simulink model "Udan_SOC"  (R2017b)
settings: Solver=FixedStepAuto  StartTime=0.0  StopTime=1000  FixedStep=0.1  RelTol=1e-3
values from neighbouring files (symbols this model uses):
  DenominatorOfIntegratorFactor = 100.0    [SOC_Stateflow.sldd]
  SOC_CalcSohLKT = 1.0    [SOC_Stateflow.sldd]
  SOC_CalcSOHTempLimit = 70.0    [SOC_Stateflow.sldd]
  SOC_CapPerCycle = 100.0    [SOC_Stateflow.sldd]
  SOC_CapTemp_HLimit = 200.0    [SOC_Stateflow.sldd]
  SOC_CapTemp_LLimit = 0.0    [SOC_Stateflow.sldd]
  Soc_ConfigInfo = 0    [SOC_Stateflow.sldd]
  SOC_DchgEndCalib = 0.0    [SOC_Stateflow.sldd]
  SOC_DiffVoltMin = 10.0    [SOC_Stateflow.sldd]
  SOC_DSOCJumpMax = 500.0    [SOC_Stateflow.sldd]
  SOC_EfficientHighLimit = 250.0    [SOC_Stateflow.sldd]
  SOC_EfficientLowLimit = 40.0    [SOC_Stateflow.sldd]
  SOC_EmptyAus = 0.0    [SOC_Stateflow.sldd]
  SOC_EnableOcv = 1.0    [SOC_Stateflow.sldd]
  SOC_END_CALIB_STATE : value not decoded    [SOC_Stateflow.sldd]
  SOC_HighRealSoc = 95.0    [SOC_Stateflow.sldd]
  SOC_LKTSohCycles = 0.0 1.0 10.0 20.0 30.0 40.0 50.0 60.0 70.0 80.0 90.0 100.0 110.0 120.0 130.0 140.0 150.0 160.0 170.0 180.0 190.0 200.0 210.0 220.0 230.0 240.0 250.0 260.0 270.0 280.0 290.0 300.0 310.0 320.0 330.0 340.0 350.0 360.0 370.0 380.0 390.0 400.0 410.0 420.0 430.0 440.0 450.0 460.0 470.0 480.0 490.0 500.0 510.0 520.0 530.0 540.0 550.0 560.0 570.0 580.0 590.0 600.0 610.0 620.0 630.0 640.0 650.0 660.0 670.0    [SOC_Stateflow.sldd]
  SOC_LKTSohTable = 1000.0 991.0 989.0 992.0 993.0 995.0 994.0 993.0 1000.0 997.0 1002.0 1000.0 992.0 1000.0 989.0 992.0 989.0 994.0 989.0 993.0 994.0 994.0 994.0 993.0 991.0 991.0 992.0 993.0 991.0 985.0 985.0 985.0 979.0 975.0 978.0 984.0 982.0 974.0 975.0 972.0 972.0 975.0 977.0 977.0 974.0 971.0 973.0 971.0 966.0 968.0 965.0 959.0 957.0 956.0 957.0 954.0 955.0 951.0 954.0 951.0 942.0 942.0 940.0 942.0 947.0 949.0    [SOC_Stateflow.sldd]
  SOC_LowRealSoc = 5.0    [SOC_Stateflow.sldd]
  SOC_NominalCap_AmS = 576000000.0    [SOC_Stateflow.sldd]
  SOC_NominalVol = 4000.0    [SOC_Stateflow.sldd]
  SOC_OCVTemp_HLimit = 106.0    [SOC_Stateflow.sldd]
  SOC_OCVTemp_LLimit = 29.0    [SOC_Stateflow.sldd]
  SOC_ShortCalibDSoc = 1.0    [SOC_Stateflow.sldd]
  SOC_SOCResolution = 10000.0    [SOC_Stateflow.sldd]
  SOC_SohCalcCapPercent = 8.0    [SOC_Stateflow.sldd]
  SOC_SohCalcHighLimit = 60.0    [SOC_Stateflow.sldd]
  SOC_SohCalcLowLimit = 10.0    [SOC_Stateflow.sldd]
  SOC_SohCalcMidLimit = 30.0    [SOC_Stateflow.sldd]
  SOC_SOHResolution = 1000.0    [SOC_Stateflow.sldd]
  SOC_State = <binary blob, 1163 chars, not shown>    [SOC_Stateflow.sldd]
  SOC_TempCap_CapBuffer : value not decoded    [SOC_Stateflow.sldd]
  SOC_TempCap_TempBuffer : value not decoded    [SOC_Stateflow.sldd]
  SocOcvCalib_ConfigInfo = 0.0    [SOC_Stateflow.sldd]
  SocOcvCalib_SocBuffer1 : value not decoded    [SOC_Stateflow.sldd]
  SocOcvCalib_TempBuffer : value not decoded    [SOC_Stateflow.sldd]
  SocOcvCalib_VoltageBuffer1 = 3300.0 3303.0 3305.0 3307.0 3310.0 3311.0 3313.0 3314.0 3316.0 3317.0 3319.0 3320.0 3322.0 3323.0 3325.0 3322.0 3323.0 3325.0 3310.0 3313.0 3315.0 3317.0 3320.0 3321.0 3323.0 3324.0 3326.0 3327.0 3329.0 3330.0 3332.0 3333.0 3335.0 3332.0 3333.0 3335.0 3320.0 3323.0 3325.0 3327.0 3330.0 3331.0 3333.0 3334.0 3336.0 3337.0 3339.0 3340.0 3342.0 3343.0 3345.0 3342.0 3343.0 3345.0 3330.0 3333.0 3335.0 3    [SOC_Stateflow.sldd]
  SOHCalibCycle = 10.0    [SOC_Stateflow.sldd]
undefined symbols (not defined in the file or in its folder): DatetimeM_GetReturnType, ParameterM_EeepParaIndexType, Soc_CumuLativeTypeType, SOC_EgthTempChgValue, Soc_EnergyBuffer, SOC_FithTempChgValue, SOC_FstSlowTempChgValue, SOC_FstTempChgValue, SOC_FthTempChgValue, SOC_MaxCap_AmS, SOC_SethTempChgValue, SOC_SixTempChgValue, SOC_SndSlowTempChgValue, SOC_SndTempChgValue, SOC_TrdSlowTempChgValue, SOC_TrdTempChgValue, SocDiagCalib_NoCalibReasonType
libraries: simulink x138, hdlsllib x24, dspindex x4
(part 1 of 10)
settings Model: DataDictionary=SOC_Stateflow.sldd  Creator=Administrator  LastModifiedBy=Administrator
settings OptimizationCC: DefaultParameterBehavior=Inlined  UseDivisionForNetSlopeComputation=on  PassReuseOutputArgsAs=Individual arguments  LifeSpan=inf
settings DebuggingCC: SignalInfNanChecking=error  IntegerOverflowMsg=error  ParameterTunabilityLossMsg=error  AssertControl=DisableAll  SFExecutionAtInitializationDiag=none
settings HardwareCC: ProdBitPerInt=16  ProdBitPerPointer=16  ProdBitPerSizeT=16  ProdBitPerPtrDiffT=16  ProdLargestAtomicFloat=None  ProdEndianess=BigEndian  ProdWordSize=16  ProdHWDeviceType=Freescale->HC(S)12
settings SFSimCC: MATLABDynamicMemAlloc=off
settings RTWCC: SystemTargetFile=ert.tlc  GenCodeOnly=on  TemplateMakefile=ert_default_tmf  GenerateReport=on  CustomSourceCode=/*lint -e* -w0 */  CustomHeaderCode=/*lint -e* -w0 */  Toolchain=MinGW64 | gmake (64-bit Windows)  IncludeHyperlinkInReport=on  GenerateTraceInfo=on  GenerateTraceReport=on  GenerateTraceReportSl=on  GenerateTraceReportSf=on  GenerateTraceReportEml=on
settings CodeAppCC: ForceParamTrailComments=on  IgnoreCustomStorageClasses=off  OperatorAnnotations=on  SimulinkDataObjDesc=on  SFDataObjDesc=on  InsertBlockDesc=on  StateflowObjectComments=on
settings ERTTargetCC: TargetLangStandard=C99 (ISO)  UtilityFuncGeneration=Shared location  SupportNonFinite=off  SupportVariableSizeSignals=on  ParenthesesLevel=Maximum  CastingMode=Standards  InlinedParameterPlacement=NonHierarchical  ERTCustomFileTemplate=example_file_process.tlc  GlobalDataDefinition=InSeparateSourceFile  DataDefinitionFile=UDAN_SOCCalibdata.c  DataReferenceFile=UDAN_SOCCalibdata.h  EnableSignedLeftShifts=off  EnableSignedRightShifts=off
settings ConfigComp: DVMaxProcessTime=30000  DVTestSuiteOptimization=CombinedObjectives (Nonlinear Extended)  DVDetectActiveLogic=on  DVDetectFloatOverflow=off  DVSaveReport=on

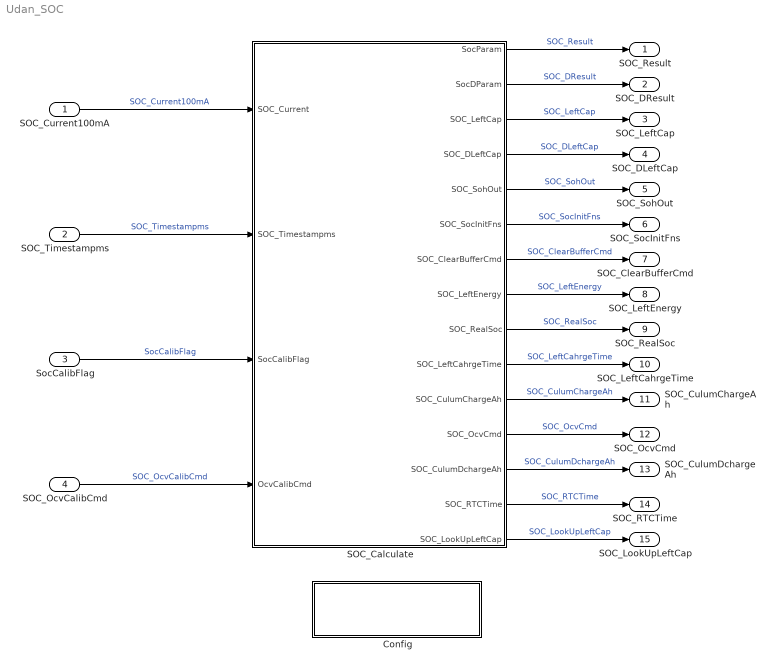
== system Udan_SOC ==
  SOC_Current100mA : Inport
  SOC_Timestampms : Inport  Port=2  OutDataTypeStr=uint32  PortDimensions=[1]
  SocCalibFlag : Inport  Port=3  OutDataTypeStr=uint8  PortDimensions=[1]
  SOC_OcvCalibCmd : Inport  Port=4
  Config : Subsystem
      mask help: 打开Ocv-Soc的电压曲线
      settings: OpenFcn=run('BlockConfig.m')
      mask Display: disp('双击完成Configuration配置')
  SOC_Calculate : Subsystem  TreatAsAtomicUnit=on  RTWFcnName=SOC_Calculate
      settings: RTWSystemCode=Nonreusable function  RTWFcnNameOpts=User specified
  SOC_Result : Outport
  SOC_DResult : Outport  Port=2
  SOC_LeftCap : Outport  Port=3
  SOC_DLeftCap : Outport  Port=4
  SOC_SohOut : Outport  Port=5
  SOC_SocInitFns : Outport  Port=6
  SOC_ClearBufferCmd : Outport  Port=7
  SOC_LeftEnergy : Outport  Port=8
  SOC_RealSoc : Outport  Port=9
  SOC_LeftCahrgeTime : Outport  Port=10
  SOC_CulumChargeAh : Outport  Port=11
  SOC_OcvCmd : Outport  Port=12
  SOC_CulumDchargeAh : Outport  Port=13
  SOC_RTCTime : Outport  Port=14
  SOC_LookUpLeftCap : Outport  Port=15
  wires:
  SOC_Calculate/1(SocParam) -> SOC_Result/1  "SOC_Result"
  SOC_Calculate/2(SocDParam) -> SOC_DResult/1  "SOC_DResult"
  SOC_Calculate/4(SOC_DLeftCap) -> SOC_DLeftCap/1  "SOC_DLeftCap"
  SOC_Calculate/3(SOC_LeftCap) -> SOC_LeftCap/1  "SOC_LeftCap"
  SOC_Current100mA/1 -> SOC_Calculate/1(SOC_Current)  "SOC_Current100mA"
  SOC_Calculate/5(SOC_SohOut) -> SOC_SohOut/1  "SOC_SohOut"
  SOC_Calculate/6(SOC_SocInitFns) -> SOC_SocInitFns/1  "SOC_SocInitFns"
  SOC_Timestampms/1 -> SOC_Calculate/2(SOC_Timestampms)  "SOC_Timestampms"
  SocCalibFlag/1 -> SOC_Calculate/3(SocCalibFlag)  "SocCalibFlag"
  SOC_Calculate/7(SOC_ClearBufferCmd) -> SOC_ClearBufferCmd/1  "SOC_ClearBufferCmd"
  SOC_Calculate/8(SOC_LeftEnergy) -> SOC_LeftEnergy/1  "SOC_LeftEnergy"
  SOC_Calculate/9(SOC_RealSoc) -> SOC_RealSoc/1  "SOC_RealSoc"
  SOC_Calculate/10(SOC_LeftCahrgeTime) -> SOC_LeftCahrgeTime/1  "SOC_LeftCahrgeTime"
  SOC_Calculate/11(SOC_CulumChargeAh) -> SOC_CulumChargeAh/1  "SOC_CulumChargeAh"
  SOC_Calculate/12(SOC_OcvCmd) -> SOC_OcvCmd/1  "SOC_OcvCmd"
  SOC_Calculate/13(SOC_CulumDchargeAh) -> SOC_CulumDchargeAh/1  "SOC_CulumDchargeAh"
  SOC_Calculate/14(SOC_RTCTime) -> SOC_RTCTime/1  "SOC_RTCTime"
  SOC_Calculate/15(SOC_LookUpLeftCap) -> SOC_LookUpLeftCap/1  "SOC_LookUpLeftCap"
  SOC_OcvCalibCmd/1 -> SOC_Calculate/4(OcvCalibCmd)  "SOC_OcvCalibCmd"

== system Udan_SOC/Config ==

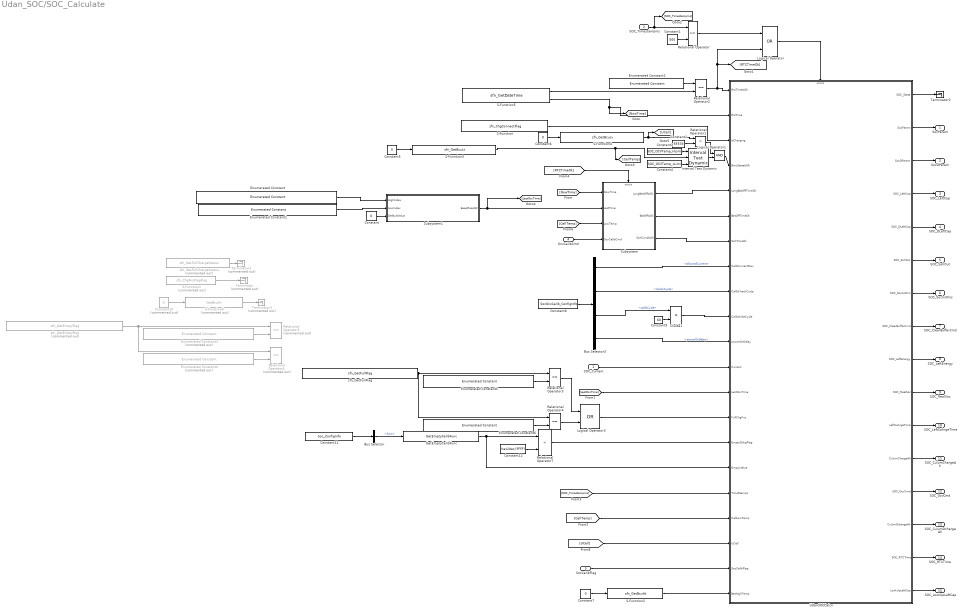
== system Udan_SOC/SOC_Calculate ==
  SOC_Current : Inport
  SOC_Timestampms : Inport  Port=2  OutDataTypeStr=uint32  PortDimensions=[1]
  SocCalibFlag : Inport  Port=3  OutDataTypeStr=uint8  PortDimensions=[1]
  OcvCalibCmd : Inport  Port=4
  Bus Selector : BusSelector  OutputSignals=func
  Bus Selector3 : BusSelector  OutputSignals=allowedCurrent,checkCycle,calibCycle,powerOnDelay
  Constant : Constant  Value=0  OutDataTypeStr=uint32
  Constant1 : Constant  Value=500  OutDataTypeStr=uint16
  Constant10 : Constant  Commented=on  Value=0  OutDataTypeStr=uint8
  Constant11 : Constant  Value=Soc_ConfigInfo  OutDataTypeStr=Bus: Soc_ConfigInfoType
  Constant12 : Constant  Value=hex2dec('FFFF')
  Constant2 : Constant  Value=65534  OutDataTypeStr=uint16
  Constant3 : Constant  Value=SOC_OCVTemp_HLimit  OutDataTypeStr=uint8
  Constant4 : Constant  Value=SOC_OCVTemp_LLimit  OutDataTypeStr=uint8
  Constant5 : Constant  Value=0  OutDataTypeStr=uint8
  Constant6 : Constant  Value=0  OutDataTypeStr=uint8
  Constant7 : Constant  Value=0  OutDataTypeStr=uint8
  Constant8 : Constant  Value=SocOcvCalib_ConfigInfo  OutDataTypeStr=Bus: SocOcvCalib_ConfigType
  Constant9 : Constant  Value=60  OutDataTypeStr=uint8
  Divide1 : Product  Inputs=**  OutDataTypeStr=uint32
  Enumerated Constant : simulink/Sources/Enumerated Constant  OutDataTypeStr=Enum: ParameterM_EeepParaIndexType  Value=ParameterM_EeepParaIndexType.PARAMETERM_EEEP_OCVSOC_TIME_HIGH_INDEX  SampleTime=inf
      settings: SourceProductName=Simulink
  Enumerated Constant1 : simulink/Sources/Enumerated Constant  OutDataTypeStr=Enum: ParameterM_EeepParaIndexType  Value=ParameterM_EeepParaIndexType.PARAMETERM_EEEP_OCVSOC_TIME_LOW_INDEX  SampleTime=inf
      settings: SourceProductName=Simulink
  Enumerated Constant2 : simulink/Sources/Enumerated Constant  OutDataTypeStr=Enum: DatetimeM_GetReturnType  Value=DatetimeM_GetReturnType.DATETIME_TRUSTY  SampleTime=inf
      settings: SourceProductName=Simulink
  Enumerated Constant3 : simulink/Sources/Enumerated Constant  Commented=on  OutDataTypeStr=Enum: SocDiagCalib_NoCalibReasonType  Value=SocDiagCalib_NoCalibReasonType.SOC_NO_CALIB_REASON_NORMAL  SampleTime=inf
      settings: SourceProductName=Simulink
  Enumerated Constant4 : simulink/Sources/Enumerated Constant  Commented=on  OutDataTypeStr=Enum: SocDiagCalib_NoCalibReasonType  Value=SocDiagCalib_NoCalibReasonType.SOC_NO_CALIB_REASON_NOT_REL  SampleTime=inf
      settings: SourceProductName=Simulink
  Enumerated Constant5 : simulink/Sources/Enumerated Constant  OutDataTypeStr=Enum: SocDiagCalib_NoCalibReasonType  Value=SocDiagCalib_NoCalibReasonType.SOC_NO_CALIB_REASON_NORMAL  SampleTime=inf
      settings: SourceProductName=Simulink
  Enumerated Constant6 : simulink/Sources/Enumerated Constant  OutDataTypeStr=Enum: SocDiagCalib_NoCalibReasonType  Value=SocDiagCalib_NoCalibReasonType.SOC_NO_CALIB_REASON_NOT_REL  SampleTime=inf
      settings: SourceProductName=Simulink
  GetEmptyCalibFunc : S-Function  FunctionName=GetEmptyCalibFunc  SFunctionDeploymentMode=off  EnableBusSupport=off  mask(Legacy Function){SFunctionSpec=uint16 y1=SOC_EmptyCalibFunc(VoidPointer u1), ShowSpec=on}
      mask prompts: ShowSpec "Display function specification"
      mask help:
      | This block allows you to call the legacy functions specified by the following Legacy Code Tool definition:
      | def.SFunctionName = 'GetEmptyCalibFunc';
      | def.OutputFcnSpec = 'uint16 y1=SOC_EmptyCalibFunc(VoidPointer u1)';
      | def.HeaderFiles = {'Soc.h'};
      mask Help: <p>This block was generated automatically by the Legacy Code Tool. For detailed help on this tool, call<a href="matlab:legacy_code('help')"> legacy_code('help')</a>.</p>
      mask Callback ShowSpec:
      | if strcmp(get_param(gcbh, 'ShowSpec'), 'on')
      |   set_param(gcbh, 'MaskDisplay', sprintf('fprintf(''%s'');', get_param(gcbh, 'SFunctionSpec')));
      | else
      |   set_param(gcbh, 'MaskDisplay', sprintf('fprintf(''%s'');', get_param(gcbh, 'FunctionName')));
      | end
      mask Display: fprintf('uint16 y1=SOC_EmptyCalibFunc(VoidPointer u1)');
  Interval Test Dynamic : simulink/Logic and Bit Operations/Interval Test Dynamic  IntervalClosedRight=off  IntervalClosedLeft=off  OutDataTypeStr=boolean
      settings: SourceProductName=Simulink  SourceProductBaseCode=SL
  Logical Operator : Logic  Operator=OR  AllPortsSameDT=off  OutDataTypeStr=boolean
  Logical Operator1 : Logic  AllPortsSameDT=off  OutDataTypeStr=boolean
  Logical Operator3 : Logic  Operator=OR  AllPortsSameDT=off  OutDataTypeStr=boolean
  Relational Operator : RelationalOperator  OutDataTypeStr=boolean  RndMeth=Simplest
  Relational Operator1 : RelationalOperator  Operator=<  OutDataTypeStr=boolean  RndMeth=Simplest
  Relational Operator2 : RelationalOperator  Operator===  OutDataTypeStr=boolean  RndMeth=Nearest
  Relational Operator3 : RelationalOperator  Operator===  OutDataTypeStr=boolean  RndMeth=Nearest
  Relational Operator4 : RelationalOperator  Operator===  OutDataTypeStr=boolean  RndMeth=Nearest
  Relational Operator5 : RelationalOperator  Commented=on  Operator===  OutDataTypeStr=boolean  RndMeth=Nearest
  Relational Operator6 : RelationalOperator  Commented=on  Operator===  OutDataTypeStr=boolean  RndMeth=Nearest
  Relational Operator7 : RelationalOperator  Operator=<  OutDataTypeStr=boolean  RndMeth=Simplest
  S-Function : S-Function  FunctionName=sfn_ChgConnectFlag  SFunctionDeploymentMode=off  EnableBusSupport=off
  S-Function1 : S-Function  Commented=on  FunctionName=sfn_ChgFnsFlagFlag  SFunctionDeploymentMode=off  EnableBusSupport=off
  S-Function2 : S-Function  FunctionName=sfn_GetBcuHt  SFunctionDeploymentMode=off  EnableBusSupport=off
  S-Function3 : S-Function  FunctionName=sfn_GetBcuLt  SFunctionDeploymentMode=off  EnableBusSupport=off
  S-Function4 : S-Function  FunctionName=sfn_GetBcuLv  SFunctionDeploymentMode=off  EnableBusSupport=off
  S-Function5 : S-Function  FunctionName=sfn_GetDateTime  SFunctionDeploymentMode=off  EnableBusSupport=off
  S-Function6 : S-Function  Commented=on  FunctionName=GetBcuHv  SFunctionDeploymentMode=off  EnableBusSupport=off
  Subsystem : Subsystem
  Subsystem1 : Subsystem  mask(ReadEeep_uint32){}
  Terminator : Terminator  Commented=on
  Terminator1 : Terminator  Commented=on
  Terminator2 : Terminator
  Terminator3 : Terminator  Commented=on
  UdanSOCCalcn : Subsystem
  sfn_GetEmptyFlag : S-Function  Commented=on  FunctionName=sfn_GetEmptyFlag  SFunctionDeploymentMode=off  EnableBusSupport=off  mask(Legacy Function){SFunctionSpec=SocDiagCalib_NoCalibReasonType y1=SocDiagCalib_GetEmptyReason(void), ShowSpec=on}
      mask prompts: ShowSpec "Display function specification"
      mask help:
      | This block allows you to call the legacy functions specified by the following Legacy Code Tool definition:
      | def.SFunctionName = 'sfn_GetEmptyFlag';
      | def.OutputFcnSpec = 'SocDiagCalib_NoCalibReasonType y1=SocDiagCalib_GetEmptyReason(void)';
      | def.HeaderFiles = {'SocDiagCalib.h'};
      mask Help: <p>This block was generated automatically by the Legacy Code Tool. For detailed help on this tool, call<a href="matlab:legacy_code('help')"> legacy_code('help')</a>.</p>
      mask Callback ShowSpec:
      | if strcmp(get_param(gcbh, 'ShowSpec'), 'on')
      |   set_param(gcbh, 'MaskDisplay', sprintf('fprintf(''%s'');', get_param(gcbh, 'SFunctionSpec')));
      | else
      |   set_param(gcbh, 'MaskDisplay', sprintf('fprintf(''%s'');', get_param(gcbh, 'FunctionName')));
      | end
      mask Display: fprintf('SocDiagCalib_NoCalibReasonType y1=SocDiagCalib_GetEmptyReason(void)');
  sfn_GetFullChargeStatus : S-Function  Commented=on  FunctionName=sfn_GetFullChargeStatus  SFunctionDeploymentMode=off  EnableBusSupport=off  mask(Legacy Function){SFunctionSpec=uint16 y1=FullCharge_GetStatus(void), ShowSpec=on}
      mask prompts: ShowSpec "Display function specification"
      mask help:
      | This block allows you to call the legacy functions specified by the following Legacy Code Tool definition:
      | def.SFunctionName = 'sfn_GetFullChargeStatus';
      | def.OutputFcnSpec = 'uint16 y1=FullCharge_GetStatus(void)';
      | def.HeaderFiles = {'FullCharge.h'};
      mask Help: <p>This block was generated automatically by the Legacy Code Tool. For detailed help on this tool, call<a href="matlab:legacy_code('help')"> legacy_code('help')</a>.</p>
      mask Callback ShowSpec:
      | if strcmp(get_param(gcbh, 'ShowSpec'), 'on')
      |   set_param(gcbh, 'MaskDisplay', sprintf('fprintf(''%s'');', get_param(gcbh, 'SFunctionSpec')));
      | else
      |   set_param(gcbh, 'MaskDisplay', sprintf('fprintf(''%s'');', get_param(gcbh, 'FunctionName')));
      | end
      mask Display: fprintf('uint16 y1=FullCharge_GetStatus(void)');
  sfn_GetFullFlag : S-Function  FunctionName=sfn_GetFullFlag  SFunctionDeploymentMode=off  EnableBusSupport=off  mask(Legacy Function){SFunctionSpec=SocDiagCalib_NoCalibReasonType y1=SocDiagCalib_GetFullReason(void), ShowSpec=on}
      mask prompts: ShowSpec "Display function specification"
      mask help:
      | This block allows you to call the legacy functions specified by the following Legacy Code Tool definition:
      | def.SFunctionName = 'sfn_GetFullFlag';
      | def.OutputFcnSpec = 'SocDiagCalib_NoCalibReasonType y1=SocDiagCalib_GetFullReason(void)';
      | def.HeaderFiles = {'SocDiagCalib.h'};
      mask Help: <p>This block was generated automatically by the Legacy Code Tool. For detailed help on this tool, call<a href="matlab:legacy_code('help')"> legacy_code('help')</a>.</p>
      mask Callback ShowSpec:
      | if strcmp(get_param(gcbh, 'ShowSpec'), 'on')
      |   set_param(gcbh, 'MaskDisplay', sprintf('fprintf(''%s'');', get_param(gcbh, 'SFunctionSpec')));
      | else
      |   set_param(gcbh, 'MaskDisplay', sprintf('fprintf(''%s'');', get_param(gcbh, 'FunctionName')));
      | end
      mask Display: fprintf('SocDiagCalib_NoCalibReasonType y1=SocDiagCalib_GetFullReason(void)');
  SocParam : Outport
  SocDParam : Outport  Port=2
  SOC_LeftCap : Outport  Port=3
  SOC_DLeftCap : Outport  Port=4
  SOC_SohOut : Outport  Port=5
  SOC_SocInitFns : Outport  Port=6
  SOC_ClearBufferCmd : Outport  Port=7
  SOC_LeftEnergy : Outport  Port=8
  SOC_RealSoc : Outport  Port=9
  SOC_LeftCahrgeTime : Outport  Port=10
  SOC_CulumChargeAh : Outport  Port=11
  SOC_OcvCmd : Outport  Port=12
  SOC_CulumDchargeAh : Outport  Port=13
  SOC_RTCTime : Outport  Port=14
  SOC_LookUpLeftCap : Outport  Port=15
  wires:
  UdanSOCCalcn/4(SOC_LeftCap) -> SOC_LeftCap/1
  Constant8/1 -> Bus Selector3/1
  [LastOcvTime] -> UdanSOCCalcn/13(LastOcvTime)
  Enumerated Constant/1 -> Subsystem1/1(HighIndex)
  Enumerated Constant4/1 -> Relational Operator6/2
  sfn_GetEmptyFlag/1 -> Relational Operator6/1, Relational Operator5/1
  Enumerated Constant3/1 -> Relational Operator5/2
  SOC_Timestampms/1 -> [SOC_Timestampms], Relational Operator/1
  Relational Operator7/1 -> UdanSOCCalcn/15(EmptyDchgFlag)
  Logical Operator3/1 -> UdanSOCCalcn/14(FullChgFns)
  Interval Test Dynamic/1 -> Logical Operator1/2
  S-Function5/2 -> UdanSOCCalcn/2(RtcTime), [NowTime]
  Relational Operator2/1 -> UdanSOCCalcn/1(RtcTimeIsOk), [RTCTimeOk], Logical Operator/2
  S-Function/1 -> UdanSOCCalcn/3(IsCharging)
  [CellTemp] -> UdanSOCCalcn/18(CellLowTemp)
  UdanSOCCalcn/2(SocParam) -> SocParam/1
  S-Function5/1 -> Relational Operator2/2
  UdanSOCCalcn/5(SOC_DLeftCap) -> SOC_DLeftCap/1
  UdanSOCCalcn/6(SOC_SohOut) -> SOC_SohOut/1
  SOC_Current/1 -> UdanSOCCalcn/12(Current)
  Bus Selector3/2 -> UdanSOCCalcn/9(CalibCheckCycle)  "<checkCycle>"
  Bus Selector3/3 -> Divide1/1  "<calibCycle>"
  Constant9/1 -> Divide1/2
  Enumerated Constant2/1 -> Relational Operator2/1
  Constant3/1 -> Interval Test Dynamic/1
  Constant4/1 -> Interval Test Dynamic/3
  Enumerated Constant1/1 -> Subsystem1/2(LowIndex)
  UdanSOCCalcn/3(SocDParam) -> SocDParam/1
  Divide1/1 -> UdanSOCCalcn/10(CalibWriteCycle)
  Bus Selector3/1 -> UdanSOCCalcn/8(CalibCurrentMax)  "<allowedCurrent>"
  S-Function3/1 -> [CellTemp], Interval Test Dynamic/2
  SocCalibFlag/1 -> UdanSOCCalcn/20(SocCalibFlag)
  Constant/1 -> Subsystem1/3(DefaultValue)
  UdanSOCCalcn/7(SOC_SocInitFns) -> SOC_SocInitFns/1
  Constant1/1 -> Relational Operator/2
  Logical Operator/1 -> UdanSOCCalcn/Enable
  Relational Operator/1 -> Logical Operator/1
  [SOC_Timestampms] -> UdanSOCCalcn/17(TimeStamps)
  [NowTime] -> Subsystem/1(NowTime)
  Subsystem/1(LongBatOffIsOk) -> UdanSOCCalcn/5(LongBatOffTimeOk)
  Subsystem/2(BatOffIsOk) -> UdanSOCCalcn/6(BatOffTimeOk)
  Subsystem/3(SohCondIsOk) -> UdanSOCCalcn/7(SohTimeOk)
  Subsystem1/1(EeepRead32) -> [LastOcvTime], Subsystem/2(LastTime)
  [RTCTimeOk] -> Subsystem/Enable
  S-Function4/1 -> [UCell], Relational Operator1/1
  Constant2/1 -> Relational Operator1/2
  Logical Operator1/1 -> UdanSOCCalcn/4(BmuStateIsOk)
  Relational Operator1/1 -> Logical Operator1/1
  [UCell] -> UdanSOCCalcn/19(UCell)
  S-Function1/1 -> Terminator/1
  Constant5/1 -> S-Function3/1
  Constant6/1 -> S-Function4/1
  Enumerated Constant5/1 -> Relational Operator3/2
  Relational Operator4/1 -> Logical Operator3/2
  sfn_GetFullFlag/1 -> Relational Operator4/1, Relational Operator3/1
  Relational Operator3/1 -> Logical Operator3/1
  sfn_GetFullChargeStatus/1 -> Terminator1/1
  Enumerated Constant6/1 -> Relational Operator4/2
  UdanSOCCalcn/8(SOC_ClearBufferCmd) -> SOC_ClearBufferCmd/1
  UdanSOCCalcn/1(SOC_State) -> Terminator2/1
  UdanSOCCalcn/9(SOC_LeftEnergy) -> SOC_LeftEnergy/1
  UdanSOCCalcn/10(SOC_RealSoc) -> SOC_RealSoc/1
  UdanSOCCalcn/11(LeftCahrgeTime) -> SOC_LeftCahrgeTime/1
  UdanSOCCalcn/12(CulumChargeAh) -> SOC_CulumChargeAh/1
  UdanSOCCalcn/13(SOC_OcvCmd) -> SOC_OcvCmd/1
  Constant7/1 -> S-Function2/1
  S-Function2/1 -> UdanSOCCalcn/21(BatHighTemp)
  UdanSOCCalcn/14(CulumDchargeAh) -> SOC_CulumDchargeAh/1
  [CellTemp] -> Subsystem/3(LowTemp)
  Constant10/1 -> S-Function6/1
  S-Function6/1 -> Terminator3/1
  Bus Selector3/4 -> UdanSOCCalcn/11(powerOnDelay)  "<powerOnDelay>"
  UdanSOCCalcn/15(SOC_RTCTime) -> SOC_RTCTime/1
  UdanSOCCalcn/16(LookUpLeftCap) -> SOC_LookUpLeftCap/1
  Bus Selector/1 -> GetEmptyCalibFunc/1  "<func>"
  GetEmptyCalibFunc/1 -> UdanSOCCalcn/16(EmptyValue), Relational Operator7/1
  Constant12/1 -> Relational Operator7/2
  Constant11/1 -> Bus Selector/1
  OcvCalibCmd/1 -> Subsystem/4(OcvCalibCmd)

== system Udan_SOC/SOC_Calculate/Subsystem ==
  NowTime : Inport
  LastTime : Inport  Port=2
  LowTemp : Inport  Port=3
  OcvCalibCmd : Inport  Port=4
  Enable : EnablePort
  Add : Sum  Inputs=+-  AccumDataTypeStr=int32  OutDataTypeStr=int32
  Bus Selector1 : BusSelector  OutputSignals=calibCycle
  Bus Selector2 : BusSelector  OutputSignals=longCycle
  Bus Selector3 : BusSelector  OutputSignals=calibCycle
  Constant : Constant  Value=1000  OutDataTypeStr=uint16
  Constant1 : Constant  Value=SOC_CalcSOHTempLimit
  Constant2 : Constant  Value=SocOcvCalib_ConfigInfo  OutDataTypeStr=Bus: SocOcvCalib_ConfigType
  Constant3 : Constant  Value=SocOcvCalib_ConfigInfo  OutDataTypeStr=Bus: SocOcvCalib_ConfigType
  Constant4 : Constant  Value=2  OutDataTypeStr=uint8
  Constant5 : Constant  Value=60  OutDataTypeStr=uint8
  Constant6 : Constant  Value=SocOcvCalib_ConfigInfo  OutDataTypeStr=Bus: SocOcvCalib_ConfigType
  Constant7 : Constant  Value=SOHCalibCycle
  Constant8 : Constant  OutDataTypeStr=uint8
  Delay1 : Delay  DelayLength=1  InitialCondition=0
  Delay10 : Delay  DelayLength=1  InitialCondition=0
  Divide : Product  Inputs=*/  OutDataTypeStr=int32
  Logical Operator{,1..3,6} (5 alike) : Logic  AllPortsSameDT=off  OutDataTypeStr=boolean
  Logical Operator4 : Logic  Operator=NOT  AllPortsSameDT=off  OutDataTypeStr=boolean
  Logical Operator5 : Logic  Operator=OR  AllPortsSameDT=off  OutDataTypeStr=boolean
  Logical Operator7 : Logic  Operator=NOT  AllPortsSameDT=off  OutDataTypeStr=boolean
  Logical Operator8 : Logic  Operator=OR  AllPortsSameDT=off  OutDataTypeStr=boolean
  Relational Operator : RelationalOperator  OutDataTypeStr=boolean  RndMeth=Simplest
  Relational Operator1 : RelationalOperator  OutDataTypeStr=boolean  RndMeth=Nearest
  Relational Operator2 : RelationalOperator  OutDataTypeStr=boolean  RndMeth=Simplest
  Relational Operator3 : RelationalOperator  OutDataTypeStr=boolean  RndMeth=Nearest
  Relational Operator4 : RelationalOperator  OutDataTypeStr=boolean  RndMeth=Nearest
  Relational Operator5 : RelationalOperator  Operator===  OutDataTypeStr=boolean  RndMeth=Simplest
  Relational Operator6 : RelationalOperator  Operator===  OutDataTypeStr=boolean  RndMeth=Simplest
  Switch : Switch  Criteria=u2 > Threshold
  LongBatOffIsOk : Outport
  BatOffIsOk : Outport  Port=2
  SohCondIsOk : Outport  Port=3
  wires:
  Relational Operator1/1 -> Logical Operator2/1
  Add/1 -> Divide/1
  NowTime/1 -> Add/1
  Relational Operator3/1 -> Logical Operator1/1
  Constant6/1 -> Bus Selector1/1
  Bus Selector2/1 -> Relational Operator1/2  "<longCycle>"
  Constant2/1 -> Bus Selector2/1
  Constant5/1 -> Divide/2
  LastTime/1 -> Relational Operator/1, Add/2
  Relational Operator4/1 -> Logical Operator/1
  Bus Selector1/1 -> Relational Operator3/2  "<calibCycle>"
  Divide/1 -> Relational Operator4/1, Relational Operator3/1, Relational Operator1/1
  Constant/1 -> Relational Operator/2
  Relational Operator/1 -> Logical Operator2/2, Logical Operator1/2, Logical Operator/2
  Logical Operator8/1 -> BatOffIsOk/1
  Logical Operator5/1 -> LongBatOffIsOk/1
  Logical Operator/1 -> SohCondIsOk/1
  Constant3/1 -> Bus Selector3/1
  Relational Operator2/1 -> Switch/2
  LowTemp/1 -> Relational Operator2/1
  Constant1/1 -> Relational Operator2/2
  Bus Selector3/1 -> Switch/3  "<calibCycle>"
  Constant7/1 -> Switch/1
  Switch/1 -> Relational Operator4/2
  Constant4/1 -> Relational Operator5/2
  Delay10/1 -> Logical Operator4/1
  Logical Operator4/1 -> Logical Operator3/2
  Relational Operator5/1 -> Delay10/1, Logical Operator3/1
  Logical Operator2/1 -> Logical Operator5/2
  Logical Operator3/1 -> Logical Operator5/1
  OcvCalibCmd/1 -> Relational Operator6/1, Relational Operator5/1
  Constant8/1 -> Relational Operator6/2
  Relational Operator6/1 -> Delay1/1, Logical Operator6/1
  Logical Operator7/1 -> Logical Operator6/2
  Delay1/1 -> Logical Operator7/1
  Logical Operator6/1 -> Logical Operator8/1
  Logical Operator1/1 -> Logical Operator8/2

== system Udan_SOC/SOC_Calculate/Subsystem1 ==
  HighIndex : Inport
  LowIndex : Inport  Port=2
  DefaultValue : Inport  Port=3
  Constant1 : Constant  Value=0  OutDataTypeStr=uint8
  Constant2 : Constant  Value=0  OutDataTypeStr=uint8
  Logical Operator : Logic  AllPortsSameDT=off  OutDataTypeStr=boolean
  Logical Operator1 : Logic  Operator=NOT  AllPortsSameDT=off  OutDataTypeStr=boolean
  Relational Operator : RelationalOperator  Operator===  OutDataTypeStr=boolean  RndMeth=Simplest
  Relational Operator1 : RelationalOperator  Operator===  OutDataTypeStr=boolean  RndMeth=Simplest
  S-Function : S-Function  FunctionName=sfn_NVMRead  SFunctionDeploymentMode=off  EnableBusSupport=off
  S-Function1 : S-Function  FunctionName=sfn_NVMRead  SFunctionDeploymentMode=off  EnableBusSupport=off
  Subsystem : Subsystem
  Switch : Switch  Criteria=u2 > Threshold
  EeepRead32 : Outport
  wires:
  DefaultValue/1 -> Switch/1
  [ReadLowOk] -> Logical Operator/1
  S-Function/2 -> Subsystem/1(HighIndex)
  S-Function/1 -> Relational Operator/1
  S-Function1/2 -> Subsystem/2(LowIndex)
  HighIndex/1 -> S-Function/1
  Constant1/1 -> Relational Operator/2
  Constant2/1 -> Relational Operator1/2
  LowIndex/1 -> S-Function1/1
  Relational Operator/1 -> Logical Operator/2
  Logical Operator/1 -> Logical Operator1/1, Subsystem/Enable
  Relational Operator1/1 -> [ReadLowOk]
  S-Function1/1 -> Relational Operator1/1
  Subsystem/1(soc) -> Switch/3
  Logical Operator1/1 -> Switch/2
  Switch/1 -> EeepRead32/1
